simulink model "TP7 MLI"  (R2023b)
settings: Solver=VariableStepAuto  StartTime=0.0  StopTime=0.1  RelTol=1e-3
libraries: spsIGBTDiodeLib x12, spsSeriesRLCBranchLib x6, spsACCurrentSourceLib x4, spsGroundLib x3, spsDCVoltageSourceLib x2, spsThreePhaseVIMeasurementLib x2, spsTriangleGeneratorLib x1, sps_lib x1
settings Model: Creator=sohayl  LastModifiedBy=sohayl

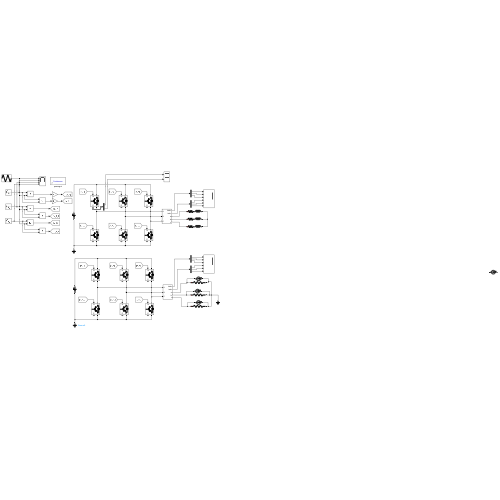
[thumbnail: Simulink's stored preview of the top-level diagram]
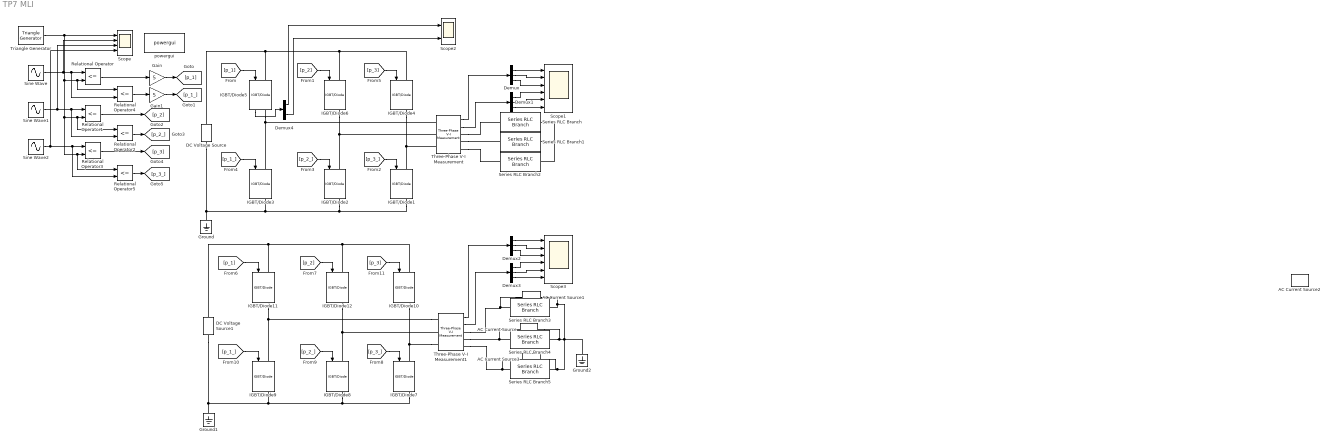
== system TP7 MLI ==
  AC Current Source : spsACCurrentSourceLib/AC Current Source  Amplitude=5  Phase=0  Frequency=50  SampleTime=0  Measurements=None
      settings: LibrarySourceBlock=sps_lib/Sources/AC Current Source
  AC Current Source1 : spsACCurrentSourceLib/AC Current Source  Amplitude=5  Phase=0  Frequency=50  SampleTime=0  Measurements=None
      settings: LibrarySourceBlock=sps_lib/Sources/AC Current Source
  AC Current Source2 : spsACCurrentSourceLib/AC Current Source  Amplitude=10  Phase=0  Frequency=60  SampleTime=0  Measurements=None
      settings: LibrarySourceBlock=sps_lib/Sources/AC Current Source
  AC Current Source3 : spsACCurrentSourceLib/AC Current Source  Amplitude=5  Phase=0  Frequency=50  SampleTime=0  Measurements=None
      settings: LibrarySourceBlock=sps_lib/Sources/AC Current Source
  DC Voltage Source : spsDCVoltageSourceLib/DC Voltage Source  Amplitude=220*sqrt(2)  Measurements=None
  DC Voltage Source1 : spsDCVoltageSourceLib/DC Voltage Source  Amplitude=220*sqrt(2)  Measurements=None
  Demux{,1..3} (4 alike) : Demux  Outputs=3
  Demux4 : Demux  Outputs=2
  Gain : Gain  Gain=5
  Gain1 : Gain  Gain=5
  Ground : spsGroundLib/Ground  LConnTagsString=a
  Ground1 : spsGroundLib/Ground  LConnTagsString=a
  Ground2 : spsGroundLib/Ground  LConnTagsString=a
  IGBT/Diode{1..12} (12 alike) : spsIGBTDiodeLib/IGBT//Diode  Ron=1e-3  Rs=1e5  Cs=inf  Measurements=on
  Relational Operator{,1..5} (6 alike) : RelationalOperator  Operator=<=  OutDataTypeStr=boolean  RndMeth=Simplest  InputSameDT=off
  Scope : Scope  NumInputPorts=4
  Scope1 : Scope  NumInputPorts=6
  Scope2 : Scope  NumInputPorts=2
  Scope3 : Scope  NumInputPorts=6
  Series RLC Branch : spsSeriesRLCBranchLib/Series RLC Branch  LConnTagsString=__new0  RConnTagsString=__new0  BranchType=RL  Resistance=1  Inductance=1e-3  SetiL0=off  InitialCurrent=0  Capacitance=1e-6  Setx0=off  InitialVoltage=0  Measurements=None
  Series RLC Branch1 : spsSeriesRLCBranchLib/Series RLC Branch  LConnTagsString=__new0  RConnTagsString=__new0  BranchType=RL  Resistance=1  Inductance=1e-3  SetiL0=off  InitialCurrent=0  Capacitance=1e-6  Setx0=off  InitialVoltage=0  Measurements=None
  Series RLC Branch2 : spsSeriesRLCBranchLib/Series RLC Branch  LConnTagsString=__new0  RConnTagsString=__new0  BranchType=RL  Resistance=1  Inductance=1e-3  SetiL0=off  InitialCurrent=0  Capacitance=1e-6  Setx0=off  InitialVoltage=0  Measurements=None
  Series RLC Branch3 : spsSeriesRLCBranchLib/Series RLC Branch  LConnTagsString=__new0  RConnTagsString=__new0  BranchType=R  Resistance=10000  Inductance=1e-3  SetiL0=off  InitialCurrent=0  Capacitance=1e-6  Setx0=off  InitialVoltage=0  Measurements=None
  Series RLC Branch4 : spsSeriesRLCBranchLib/Series RLC Branch  LConnTagsString=__new0  RConnTagsString=__new0  BranchType=R  Resistance=10000  Inductance=1e-3  SetiL0=off  InitialCurrent=0  Capacitance=1e-6  Setx0=off  InitialVoltage=0  Measurements=None
  Series RLC Branch5 : spsSeriesRLCBranchLib/Series RLC Branch  LConnTagsString=__new0  RConnTagsString=__new0  BranchType=R  Resistance=10000  Inductance=1e-3  SetiL0=off  InitialCurrent=0  Capacitance=1e-6  Setx0=off  InitialVoltage=0  Measurements=None
  Sine Wave : Sin  Frequency=50  SampleTime=0
  Sine Wave1 : Sin  Frequency=50  Phase=2*pi/3  SampleTime=0
  Sine Wave2 : Sin  Frequency=50  Phase=4*pi/3  SampleTime=0
  Three-Phase V-I Measurement : spsThreePhaseVIMeasurementLib/Three-Phase V-I Measurement  VoltageMeasurement=phase-to-ground  SetLabelV=off  LabelV=Vabc  Vpu=off  VpuLL=off  CurrentMeasurement=yes  SetLabelI=off  LabelI=Iabc  Ipu=off  Pbase=100e6  Vbase=500e3  OutputType=Complex  PhasorSimulation=off  PSBequivalent=0
  Three-Phase V-I Measurement1 : spsThreePhaseVIMeasurementLib/Three-Phase V-I Measurement  VoltageMeasurement=phase-to-ground  SetLabelV=off  LabelV=Vabc  Vpu=off  VpuLL=off  CurrentMeasurement=yes  SetLabelI=off  LabelI=Iabc  Ipu=off  Pbase=100e6  Vbase=500e3  OutputType=Complex  PhasorSimulation=off  PSBequivalent=0
  Triangle Generator : spsTriangleGeneratorLib/Triangle Generator  Freq=60*6  Phase=90  Ts=0
  powergui : sps_lib/powergui  Priority=1  SimulationMode=Continuous  SampleTime=50e-6  frequency=60  Iterations=50  frequencyindice=0  Pbase=100e6  ErrMax=1e-4  UnitsV=kV  UnitsW=MW  buscounter=0  FunctionMessages=off  echomessages=off  EnableUseOfTLC=off  CurrentSourceSwitches=off  DisableSnubberDevices=off  DisableRonSwitches=off  DisableVfSwitches=off  DisplayEquations=off  AutomaticDiscreteSolvers=off  SolverType=Tustin/Backward Euler (TBE)  Interpol=off  ExternalGateDelay=off  methode=off  Ts=100  x0status=blocks  SPID=on  SwTol=0  HookPort=off  NonlinearTolerance=1e-4  nMaxIteration=100  ContinueOnMaxIteration=off  RestoreLinks=warning  ResistiveCurrentMeasurement=off  Frange=[0:2:500]  Ylog=off  Xlog=on  ShowGrid=off  save=off  variable=ZData  structure=0  ZoomFFT=off  StartTime=0.0  cycles=1  DisplayStyle=1  fundamental=60  FreqAxis=off  MaxFrequency=1000  frequencyindicesteady=1  RmsSteady=1  display=off
  wires:
  Sine Wave2/1 -> Scope/4, Relational Operator5/2, Relational Operator3/1
  Sine Wave1/1 -> Scope/3, Relational Operator2/2, Relational Operator1/1
  Sine Wave/1 -> Scope/2, Relational Operator4/2, Relational Operator/1
  Triangle Generator/1 -> Relational Operator5/1, Relational Operator3/2, Relational Operator2/1, Relational Operator1/2, Relational Operator4/1, Relational Operator/2, Scope/1
  Relational Operator1/1 -> [p_2]
  Relational Operator2/1 -> [p_2_]
  Relational Operator3/1 -> [p_3]
  Relational Operator5/1 -> [p_3_]
  [p_1] -> IGBT/Diode5/1
  [p_2] -> IGBT/Diode6/1
  [p_3] -> IGBT/Diode4/1
  [p_1_] -> IGBT/Diode3/1
  [p_2_] -> IGBT/Diode2/1
  [p_3_] -> IGBT/Diode1/1
  Three-Phase V-I Measurement/1 -> Demux/1
  Three-Phase V-I Measurement/2 -> Demux1/1
  Demux/1 -> Scope1/1
  Demux/2 -> Scope1/2
  Demux/3 -> Scope1/3
  Demux1/1 -> Scope1/4
  Demux1/2 -> Scope1/5
  Demux1/3 -> Scope1/6
  [p_3] -> IGBT/Diode10/1
  [p_1] -> IGBT/Diode11/1
  Demux2/1 -> Scope3/1
  Three-Phase V-I Measurement1/1 -> Demux2/1
  [p_3_] -> IGBT/Diode7/1
  Demux2/3 -> Scope3/3
  Demux2/2 -> Scope3/2
  [p_2_] -> IGBT/Diode8/1
  Demux3/2 -> Scope3/5
  Demux3/3 -> Scope3/6
  Three-Phase V-I Measurement1/2 -> Demux3/1
  Demux3/1 -> Scope3/4
  [p_2] -> IGBT/Diode12/1
  [p_1_] -> IGBT/Diode9/1
  Relational Operator/1 -> Gain/1
  Gain/1 -> [p_1]
  Relational Operator4/1 -> Gain1/1
  Gain1/1 -> [p_1_]
  IGBT/Diode5/1 -> Demux4/1
  Demux4/1 -> Scope2/1
  Demux4/2 -> Scope2/2
  connections:
  IGBT/Diode5/RConn1 -- IGBT/Diode3/LConn1 -- Three-Phase V-I Measurement/LConn1
  IGBT/Diode6/RConn1 -- Three-Phase V-I Measurement/LConn2 -- IGBT/Diode2/LConn1
  IGBT/Diode4/RConn1 -- IGBT/Diode1/LConn1 -- Three-Phase V-I Measurement/LConn3
  IGBT/Diode5/LConn1 -- IGBT/Diode4/LConn1 -- IGBT/Diode6/LConn1 -- DC Voltage Source/RConn1
  DC Voltage Source/LConn1 -- Ground/LConn1 -- IGBT/Diode1/RConn1 -- IGBT/Diode2/RConn1 -- IGBT/Diode3/RConn1
  Series RLC Branch/RConn1 -- Series RLC Branch1/RConn1 -- Series RLC Branch2/RConn1
  Three-Phase V-I Measurement/RConn1 -- Series RLC Branch/LConn1
  Three-Phase V-I Measurement/RConn2 -- Series RLC Branch1/LConn1
  Three-Phase V-I Measurement/RConn3 -- Series RLC Branch2/LConn1
  IGBT/Diode9/RConn1 -- Ground1/LConn1 -- DC Voltage Source1/LConn1 -- IGBT/Diode7/RConn1 -- IGBT/Diode8/RConn1
  Three-Phase V-I Measurement1/LConn1 -- IGBT/Diode11/RConn1 -- IGBT/Diode9/LConn1
  Ground2/LConn1 -- AC Current Source1/RConn1 -- Series RLC Branch3/RConn1 -- Series RLC Branch4/RConn1 -- AC Current Source/RConn1 -- AC Current Source3/RConn1 -- Series RLC Branch5/RConn1
  IGBT/Diode12/LConn1 -- IGBT/Diode10/LConn1 -- DC Voltage Source1/RConn1 -- IGBT/Diode11/LConn1
  IGBT/Diode12/RConn1 -- Three-Phase V-I Measurement1/LConn2 -- IGBT/Diode8/LConn1
  Three-Phase V-I Measurement1/LConn3 -- IGBT/Diode10/RConn1 -- IGBT/Diode7/LConn1
  Three-Phase V-I Measurement1/RConn2 -- AC Current Source/LConn1 -- Series RLC Branch4/LConn1
  Three-Phase V-I Measurement1/RConn1 -- AC Current Source1/LConn1 -- Series RLC Branch3/LConn1
  Three-Phase V-I Measurement1/RConn3 -- AC Current Source3/LConn1 -- Series RLC Branch5/LConn1
